simulink model "Control_Logic_b_chk2"  (R2019b)
settings: Solver=VariableStepAuto  StartTime=Start_time  StopTime=Stop_time  RelTol=1e-3
values from neighbouring files (symbols this model uses):
  Aset_N1 = 2    [Parameter_control.m]
  Aset_N10 = -10    [Parameter_control.m]
  Aset_N11 = 10    [Parameter_control.m]
  Aset_N12 = 20    [Parameter_control.m]
  Aset_N2 = 30    [Parameter_control.m]
  Aset_N3 = 3    [Parameter_control.m]
  Aset_N4 = 5    [Parameter_control.m]
  Aset_N5 = 1    [Parameter_control.m]
  Aset_N6 = 0    [Parameter_control.m]
  Aset_N7 = 0.01    [Parameter_control.m]
  Aset_N8 = 2    [Parameter_control.m]
  Aset_N9 = 0.1    [Parameter_control.m]
  Dset_N1 = 1    [Parameter_control.m]
  Dset_N2 = 1    [Parameter_control.m]
  Sample_time = 0.1    [main.m]    (also in test_tool_initialize.m)
undefined symbols (not defined in the file or in its folder): DiscIntNeverNeededParam
(part 2 of 3)

== system Control_Logic_b_chk2/OSHOTC5 ==
  In1 : Inport
  In2 : Inport  Port=2
  In3 : Inport  Port=3
  Data Type Conversion : DataTypeConversion  OutDataTypeStr=boolean
  MATLAB Function : MATLAB Function  TreatAsAtomicUnit=on  SystemSampleTime=Sample_time
  Memory : Memory  InheritSampleTime=on
  Memory1 : Memory  InheritSampleTime=on  LinearizeAsDelay=on
  Mux : Mux  Inputs=2
  Out1 : Outport  VectorParamsAs1DForOutWhenUnconnected=off
  wires:
  Memory/1 -> Mux/2
  MATLAB Function/1(y) -> Out1/1, Memory1/1
  In2/1 -> MATLAB Function/3(set)
  Mux/1 -> MATLAB Function/4(timc)
  In1/1 -> MATLAB Function/1(u)
  Memory1/1 -> Data Type Conversion/1
  Data Type Conversion/1 -> MATLAB Function/2(yold)
  MATLAB Function/2(w) -> Memory/1
  In3/1 -> Mux/1

== system Control_Logic_b_chk2/OSHOTC6 ==
  In1 : Inport
  In2 : Inport  Port=2
  In3 : Inport  Port=3
  Data Type Conversion : DataTypeConversion  OutDataTypeStr=boolean
  MATLAB Function : MATLAB Function  TreatAsAtomicUnit=on  SystemSampleTime=Sample_time
  Memory : Memory  InheritSampleTime=on
  Memory1 : Memory  InheritSampleTime=on  LinearizeAsDelay=on
  Mux : Mux  Inputs=2
  Out1 : Outport  VectorParamsAs1DForOutWhenUnconnected=off
  wires:
  Memory/1 -> Mux/2
  MATLAB Function/1(y) -> Out1/1, Memory1/1
  In2/1 -> MATLAB Function/3(set)
  Mux/1 -> MATLAB Function/4(timc)
  In1/1 -> MATLAB Function/1(u)
  Memory1/1 -> Data Type Conversion/1
  Data Type Conversion/1 -> MATLAB Function/2(yold)
  MATLAB Function/2(w) -> Memory/1
  In3/1 -> Mux/1

== system Control_Logic_b_chk2/OSHOTC7 ==
  In1 : Inport
  In2 : Inport  Port=2
  In3 : Inport  Port=3
  Data Type Conversion : DataTypeConversion  OutDataTypeStr=boolean
  MATLAB Function : MATLAB Function  TreatAsAtomicUnit=on  SystemSampleTime=Sample_time
  Memory : Memory  InheritSampleTime=on
  Memory1 : Memory  InheritSampleTime=on  LinearizeAsDelay=on
  Mux : Mux  Inputs=2
  Out1 : Outport  VectorParamsAs1DForOutWhenUnconnected=off
  wires:
  Memory/1 -> Mux/2
  MATLAB Function/1(y) -> Out1/1, Memory1/1
  In2/1 -> MATLAB Function/3(set)
  Mux/1 -> MATLAB Function/4(timc)
  In1/1 -> MATLAB Function/1(u)
  Memory1/1 -> Data Type Conversion/1
  Data Type Conversion/1 -> MATLAB Function/2(yold)
  MATLAB Function/2(w) -> Memory/1
  In3/1 -> Mux/1

== system Control_Logic_b_chk2/OSHOTC8 ==
  In1 : Inport
  In2 : Inport  Port=2
  In3 : Inport  Port=3
  Data Type Conversion : DataTypeConversion  OutDataTypeStr=boolean
  MATLAB Function : MATLAB Function  TreatAsAtomicUnit=on  SystemSampleTime=Sample_time
  Memory : Memory  InheritSampleTime=on
  Memory1 : Memory  InheritSampleTime=on  LinearizeAsDelay=on
  Mux : Mux  Inputs=2
  Out1 : Outport  VectorParamsAs1DForOutWhenUnconnected=off
  wires:
  Memory/1 -> Mux/2
  MATLAB Function/1(y) -> Out1/1, Memory1/1
  In2/1 -> MATLAB Function/3(set)
  Mux/1 -> MATLAB Function/4(timc)
  In1/1 -> MATLAB Function/1(u)
  Memory1/1 -> Data Type Conversion/1
  Data Type Conversion/1 -> MATLAB Function/2(yold)
  MATLAB Function/2(w) -> Memory/1
  In3/1 -> Mux/1

== system Control_Logic_b_chk2/OSHOTC9 ==
  In1 : Inport
  In2 : Inport  Port=2
  In3 : Inport  Port=3
  Data Type Conversion : DataTypeConversion  OutDataTypeStr=boolean
  MATLAB Function : MATLAB Function  TreatAsAtomicUnit=on  SystemSampleTime=Sample_time
  Memory : Memory  InheritSampleTime=on
  Memory1 : Memory  InheritSampleTime=on  LinearizeAsDelay=on
  Mux : Mux  Inputs=2
  Out1 : Outport  VectorParamsAs1DForOutWhenUnconnected=off
  wires:
  Memory/1 -> Mux/2
  MATLAB Function/1(y) -> Out1/1, Memory1/1
  In2/1 -> MATLAB Function/3(set)
  Mux/1 -> MATLAB Function/4(timc)
  In1/1 -> MATLAB Function/1(u)
  Memory1/1 -> Data Type Conversion/1
  Data Type Conversion/1 -> MATLAB Function/2(yold)
  MATLAB Function/2(w) -> Memory/1
  In3/1 -> Mux/1

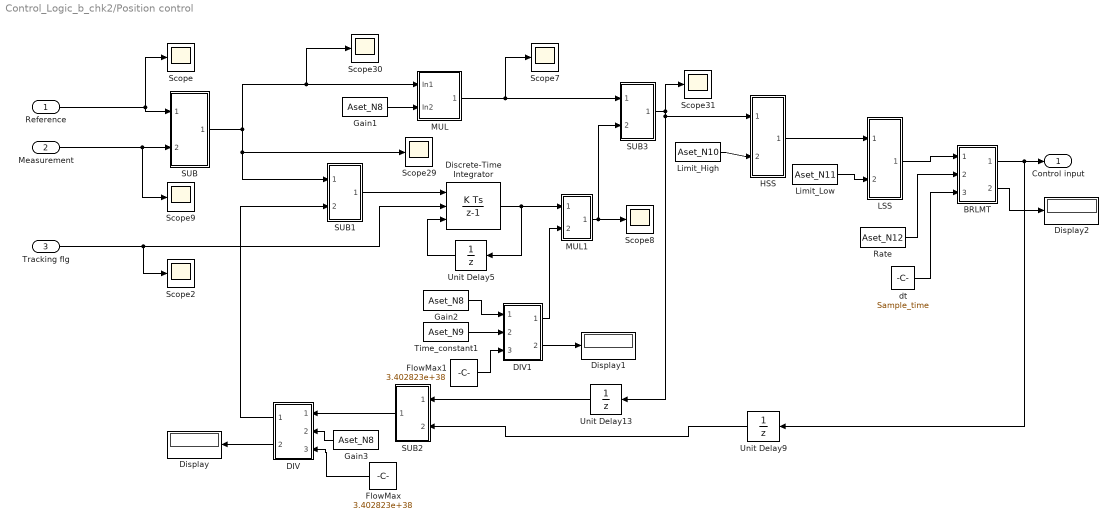
== system Control_Logic_b_chk2/Position control ==
  Reference : Inport
  Measurement : Inport  Port=2
  Tracking flg : Inport  Port=3
  BRLMT : Subsystem
  DIV : Subsystem
  DIV1 : Subsystem
  Discrete-Time Integrator : DiscreteIntegrator  ExternalReset=level  InitialConditionSource=external  SampleTime=Sample_time  ICPrevOutput=DiscIntNeverNeededParam  ICPrevScaledInput=DiscIntNeverNeededParam
  Display : Display
  Display1 : Display
  Display2 : Display
  FlowMax : Constant  Value=3.402823e+38  OutDataTypeStr=double  SampleTime=Sample_time
  FlowMax1 : Constant  Value=3.402823e+38  OutDataTypeStr=double  SampleTime=Sample_time
  Gain1 : Constant  Value=Aset_N8  OutDataTypeStr=double  SampleTime=Sample_time
  Gain2 : Constant  Value=Aset_N8  OutDataTypeStr=double  SampleTime=Sample_time
  Gain3 : Constant  Value=Aset_N8  OutDataTypeStr=double  SampleTime=Sample_time
  HSS : Subsystem
  LSS : Subsystem
  Limit_High : Constant  Value=Aset_N10  OutDataTypeStr=double  SampleTime=Sample_time
  Limit_Low : Constant  Value=Aset_N11  OutDataTypeStr=double  SampleTime=Sample_time
  MUL : Subsystem
  MUL1 : Subsystem
  Rate : Constant  Value=Aset_N12  OutDataTypeStr=double  SampleTime=Sample_time
  SUB : Subsystem
  SUB1 : Subsystem
  SUB2 : Subsystem
  SUB3 : Subsystem
  Scope{,2,7..9,29..31} (8 alike) : Scope
  Time_constant1 : Constant  Value=Aset_N9  OutDataTypeStr=double  SampleTime=Sample_time
  Unit Delay13 : UnitDelay  SampleTime=Sample_time  HasFrameUpgradeWarning=on
  Unit Delay5 : UnitDelay  SampleTime=Sample_time  HasFrameUpgradeWarning=on
  Unit Delay9 : UnitDelay  SampleTime=Sample_time  HasFrameUpgradeWarning=on
  dt : Constant  Value=Sample_time  OutDataTypeStr=double  SampleTime=Sample_time
  Control input : Outport  VectorParamsAs1DForOutWhenUnconnected=off
  wires:
  SUB3/1(Out1) -> Unit Delay13/1, HSS/1(In1), Scope31/1
  Measurement/1 -> Scope9/1, SUB/2(In2)
  SUB/1(Out1) -> Scope30/1, MUL/1(In1), SUB1/1(In1), Scope29/1
  DIV1/1(Out1) -> MUL1/2(In2)
  Unit Delay13/1 -> SUB2/1(In1)
  MUL/1(Out1) -> SUB3/1(In1), Scope7/1
  SUB2/1(Out1) -> DIV/1(In1)
  SUB1/1(Out1) -> Discrete-Time Integrator/1
  Gain1/1 -> MUL/2(In2)
  LSS/1(Out1) -> BRLMT/1(In1)
  Reference/1 -> SUB/1(In1), Scope/1
  Gain3/1 -> DIV/2(In2)
  Limit_Low/1 -> LSS/2(In2)
  Unit Delay5/1 -> Discrete-Time Integrator/3
  Tracking flg/1 -> Scope2/1, Discrete-Time Integrator/2
  Discrete-Time Integrator/1 -> MUL1/1(In1), Unit Delay5/1
  Limit_High/1 -> HSS/2(In2)
  MUL1/1(Out1) -> SUB3/2(In2), Scope8/1
  BRLMT/1(Out1) -> Control input/1, Unit Delay9/1
  Time_constant1/1 -> DIV1/2(In2)
  Gain2/1 -> DIV1/1(In1)
  HSS/1(Out1) -> LSS/1(In1)
  DIV/1(Out1) -> SUB1/2(In2)
  Unit Delay9/1 -> SUB2/2(In2)
  FlowMax/1 -> DIV/3(In3)
  DIV/2(Out2) -> Display/1
  FlowMax1/1 -> DIV1/3(In3)
  DIV1/2(Out2) -> Display1/1
  dt/1 -> BRLMT/3(In3)
  Rate/1 -> BRLMT/2(In2)
  BRLMT/2(Out2) -> Display2/1

== system Control_Logic_b_chk2/SUB ==
  In1 : Inport
  In2 : Inport  Port=2
  MATLAB Function : MATLAB Function  TreatAsAtomicUnit=on  SystemSampleTime=Sample_time
  Mux : Mux  Inputs=2
  Out1 : Outport  VectorParamsAs1DForOutWhenUnconnected=off
  wires:
  In2/1 -> Mux/2
  MATLAB Function/1(y) -> Out1/1
  Mux/1 -> MATLAB Function/1(u)
  In1/1 -> Mux/1

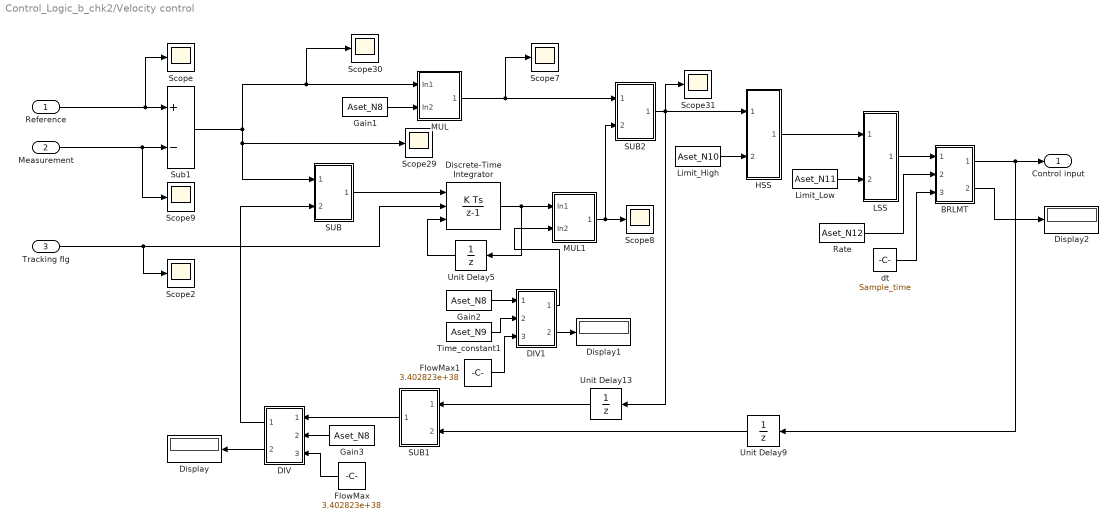
== system Control_Logic_b_chk2/Velocity control ==
  Reference : Inport
  Measurement : Inport  Port=2
  Tracking flg : Inport  Port=3
  BRLMT : Subsystem
  DIV : Subsystem
  DIV1 : Subsystem
  Discrete-Time Integrator : DiscreteIntegrator  ExternalReset=level  InitialConditionSource=external  SampleTime=Sample_time  ICPrevOutput=DiscIntNeverNeededParam  ICPrevScaledInput=DiscIntNeverNeededParam
  Display : Display
  Display1 : Display
  Display2 : Display
  FlowMax : Constant  Value=3.402823e+38  OutDataTypeStr=double  SampleTime=Sample_time
  FlowMax1 : Constant  Value=3.402823e+38  OutDataTypeStr=double  SampleTime=Sample_time
  Gain1 : Constant  Value=Aset_N8  OutDataTypeStr=double  SampleTime=Sample_time
  Gain2 : Constant  Value=Aset_N8  OutDataTypeStr=double  SampleTime=Sample_time
  Gain3 : Constant  Value=Aset_N8  OutDataTypeStr=double  SampleTime=Sample_time
  HSS : Subsystem
  LSS : Subsystem
  Limit_High : Constant  Value=Aset_N10  OutDataTypeStr=double  SampleTime=Sample_time
  Limit_Low : Constant  Value=Aset_N11  OutDataTypeStr=double  SampleTime=Sample_time
  MUL : Subsystem
  MUL1 : Subsystem
  Rate : Constant  Value=Aset_N12  OutDataTypeStr=double  SampleTime=Sample_time
  SUB : Subsystem
  SUB1 : Subsystem
  SUB2 : Subsystem
  Scope{,2,7..9,29..31} (8 alike) : Scope
  Sub1 : Sum  Inputs=+-  OutDataTypeStr=double
  Time_constant1 : Constant  Value=Aset_N9  OutDataTypeStr=double  SampleTime=Sample_time
  Unit Delay13 : UnitDelay  SampleTime=Sample_time  HasFrameUpgradeWarning=on
  Unit Delay5 : UnitDelay  SampleTime=Sample_time  HasFrameUpgradeWarning=on
  Unit Delay9 : UnitDelay  SampleTime=Sample_time  HasFrameUpgradeWarning=on
  dt : Constant  Value=Sample_time  OutDataTypeStr=double  SampleTime=Sample_time
  Control input : Outport  VectorParamsAs1DForOutWhenUnconnected=off
  wires:
  Unit Delay9/1 -> SUB1/2(In2)
  DIV/1(Out1) -> SUB/2(In2)
  HSS/1(Out1) -> LSS/1(In1)
  Gain2/1 -> DIV1/1(In1)
  Time_constant1/1 -> DIV1/2(In2)
  BRLMT/1(Out1) -> Control input/1, Unit Delay9/1
  MUL1/1(Out1) -> Scope8/1, SUB2/2(In2)
  Limit_High/1 -> HSS/2(In2)
  Discrete-Time Integrator/1 -> MUL1/1(In1), Unit Delay5/1
  Tracking flg/1 -> Discrete-Time Integrator/2, Scope2/1
  Unit Delay5/1 -> Discrete-Time Integrator/3
  Limit_Low/1 -> LSS/2(In2)
  Gain3/1 -> DIV/2(In2)
  Reference/1 -> Sub1/1, Scope/1
  LSS/1(Out1) -> BRLMT/1(In1)
  Gain1/1 -> MUL/2(In2)
  SUB/1(Out1) -> Discrete-Time Integrator/1
  SUB1/1(Out1) -> DIV/1(In1)
  MUL/1(Out1) -> SUB2/1(In1), Scope7/1
  Unit Delay13/1 -> SUB1/1(In1)
  DIV1/1(Out1) -> MUL1/2(In2)
  Sub1/1 -> SUB/1(In1), Scope29/1, MUL/1(In1), Scope30/1
  Measurement/1 -> Sub1/2, Scope9/1
  SUB2/1(Out1) -> HSS/1(In1), Scope31/1, Unit Delay13/1
  FlowMax/1 -> DIV/3(In3)
  DIV/2(Out2) -> Display/1
  DIV1/2(Out2) -> Display1/1
  FlowMax1/1 -> DIV1/3(In3)
  dt/1 -> BRLMT/3(In3)
  BRLMT/2(Out2) -> Display2/1
  Rate/1 -> BRLMT/2(In2)

== system Control_Logic_b_chk2/Position control/BRLMT ==
  In1 : Inport
  In2 : Inport  Port=2
  In3 : Inport  Port=3
  MATLAB Function : MATLAB Function  TreatAsAtomicUnit=on  SystemSampleTime=Sample_time
  Memory : Memory  InheritSampleTime=on
  Mux : Mux  Inputs=2
  Out1 : Outport  VectorParamsAs1DForOutWhenUnconnected=off
  Out2 : Outport  Port=2  VectorParamsAs1DForOutWhenUnconnected=off
  wires:
  In3/1 -> Mux/2
  In2/1 -> Mux/1
  Mux/1 -> MATLAB Function/3(set)
  MATLAB Function/2(delta) -> Out2/1
  Memory/1 -> MATLAB Function/2(yold)
  MATLAB Function/1(y) -> Out1/1, Memory/1
  In1/1 -> MATLAB Function/1(u)

== system Control_Logic_b_chk2/Position control/DIV ==
  In1 : Inport
  In2 : Inport  Port=2
  In3 : Inport  Port=3
  MATLAB Function : MATLAB Function  TreatAsAtomicUnit=on  SystemSampleTime=Sample_time
  Mux : Mux  Inputs=2
  Out1 : Outport  VectorParamsAs1DForOutWhenUnconnected=off
  Out2 : Outport  Port=2  VectorParamsAs1DForOutWhenUnconnected=off
  wires:
  In2/1 -> Mux/2
  In3/1 -> MATLAB Function/2(set)
  Mux/1 -> MATLAB Function/1(u)
  MATLAB Function/1(y) -> Out1/1
  MATLAB Function/2(err) -> Out2/1
  In1/1 -> Mux/1

== system Control_Logic_b_chk2/Position control/DIV1 ==
  In1 : Inport
  In2 : Inport  Port=2
  In3 : Inport  Port=3
  MATLAB Function : MATLAB Function  TreatAsAtomicUnit=on  SystemSampleTime=Sample_time
  Mux : Mux  Inputs=2
  Out1 : Outport  VectorParamsAs1DForOutWhenUnconnected=off
  Out2 : Outport  Port=2  VectorParamsAs1DForOutWhenUnconnected=off
  wires:
  In2/1 -> Mux/2
  In3/1 -> MATLAB Function/2(set)
  Mux/1 -> MATLAB Function/1(u)
  MATLAB Function/1(y) -> Out1/1
  MATLAB Function/2(err) -> Out2/1
  In1/1 -> Mux/1

== system Control_Logic_b_chk2/Position control/HSS ==
  In1 : Inport
  In2 : Inport  Port=2
  MATLAB Function : MATLAB Function  TreatAsAtomicUnit=on
  Mux : Mux  Inputs=2
  Out1 : Outport  VectorParamsAs1DForOutWhenUnconnected=off
  wires:
  Mux/1 -> MATLAB Function/1(u)
  In1/1 -> Mux/1
  MATLAB Function/1(y) -> Out1/1
  In2/1 -> Mux/2

== system Control_Logic_b_chk2/Position control/LSS ==
  In1 : Inport
  In2 : Inport  Port=2
  MATLAB Function : MATLAB Function  TreatAsAtomicUnit=on  SystemSampleTime=Sample_time
  Mux : Mux  Inputs=2
  Out1 : Outport  VectorParamsAs1DForOutWhenUnconnected=off
  wires:
  MATLAB Function/1(y) -> Out1/1
  Mux/1 -> MATLAB Function/1(u)
  In1/1 -> Mux/1
  In2/1 -> Mux/2

== system Control_Logic_b_chk2/Position control/MUL ==
  In1 : Inport
  In2 : Inport  Port=2
  MATLAB Function : MATLAB Function  TreatAsAtomicUnit=on  SystemSampleTime=Sample_time
  Mux : Mux  Inputs=2
  Out1 : Outport  VectorParamsAs1DForOutWhenUnconnected=off
  wires:
  Mux/1 -> MATLAB Function/1(u)
  In1/1 -> Mux/1
  In2/1 -> Mux/2
  MATLAB Function/1(y) -> Out1/1

== system Control_Logic_b_chk2/Position control/MUL1 ==
  In1 : Inport
  In2 : Inport  Port=2
  MATLAB Function : MATLAB Function  TreatAsAtomicUnit=on  SystemSampleTime=Sample_time
  Mux : Mux  Inputs=2
  Out1 : Outport  VectorParamsAs1DForOutWhenUnconnected=off
  wires:
  Mux/1 -> MATLAB Function/1(u)
  In1/1 -> Mux/1
  In2/1 -> Mux/2
  MATLAB Function/1(y) -> Out1/1

== system Control_Logic_b_chk2/Position control/SUB ==
  In1 : Inport
  In2 : Inport  Port=2
  MATLAB Function : MATLAB Function  TreatAsAtomicUnit=on  SystemSampleTime=Sample_time
  Mux : Mux  Inputs=2
  Out1 : Outport  VectorParamsAs1DForOutWhenUnconnected=off
  wires:
  In2/1 -> Mux/2
  MATLAB Function/1(y) -> Out1/1
  Mux/1 -> MATLAB Function/1(u)
  In1/1 -> Mux/1

== system Control_Logic_b_chk2/Position control/SUB1 ==
  In1 : Inport
  In2 : Inport  Port=2
  MATLAB Function : MATLAB Function  TreatAsAtomicUnit=on  SystemSampleTime=Sample_time
  Mux : Mux  Inputs=2
  Out1 : Outport  VectorParamsAs1DForOutWhenUnconnected=off
  wires:
  In2/1 -> Mux/2
  MATLAB Function/1(y) -> Out1/1
  Mux/1 -> MATLAB Function/1(u)
  In1/1 -> Mux/1

== system Control_Logic_b_chk2/Position control/SUB2 ==
  In1 : Inport
  In2 : Inport  Port=2
  MATLAB Function : MATLAB Function  TreatAsAtomicUnit=on  SystemSampleTime=Sample_time
  Mux : Mux  Inputs=2
  Out1 : Outport  VectorParamsAs1DForOutWhenUnconnected=off
  wires:
  In2/1 -> Mux/2
  MATLAB Function/1(y) -> Out1/1
  Mux/1 -> MATLAB Function/1(u)
  In1/1 -> Mux/1

== system Control_Logic_b_chk2/Position control/SUB3 ==
  In1 : Inport
  In2 : Inport  Port=2
  MATLAB Function : MATLAB Function  TreatAsAtomicUnit=on  SystemSampleTime=Sample_time
  Mux : Mux  Inputs=2
  Out1 : Outport  VectorParamsAs1DForOutWhenUnconnected=off
  wires:
  In2/1 -> Mux/2
  MATLAB Function/1(y) -> Out1/1
  Mux/1 -> MATLAB Function/1(u)
  In1/1 -> Mux/1

== system Control_Logic_b_chk2/Velocity control/BRLMT ==
  In1 : Inport
  In2 : Inport  Port=2
  In3 : Inport  Port=3
  MATLAB Function : MATLAB Function  TreatAsAtomicUnit=on  SystemSampleTime=Sample_time
  Memory : Memory  InheritSampleTime=on
  Mux : Mux  Inputs=2
  Out1 : Outport  VectorParamsAs1DForOutWhenUnconnected=off
  Out2 : Outport  Port=2  VectorParamsAs1DForOutWhenUnconnected=off
  wires:
  In3/1 -> Mux/2
  In2/1 -> Mux/1
  Mux/1 -> MATLAB Function/3(set)
  MATLAB Function/2(delta) -> Out2/1
  Memory/1 -> MATLAB Function/2(yold)
  MATLAB Function/1(y) -> Out1/1, Memory/1
  In1/1 -> MATLAB Function/1(u)

== system Control_Logic_b_chk2/Velocity control/DIV ==
  In1 : Inport
  In2 : Inport  Port=2
  In3 : Inport  Port=3
  MATLAB Function : MATLAB Function  TreatAsAtomicUnit=on  SystemSampleTime=Sample_time
  Mux : Mux  Inputs=2
  Out1 : Outport  VectorParamsAs1DForOutWhenUnconnected=off
  Out2 : Outport  Port=2  VectorParamsAs1DForOutWhenUnconnected=off
  wires:
  In2/1 -> Mux/2
  In3/1 -> MATLAB Function/2(set)
  Mux/1 -> MATLAB Function/1(u)
  MATLAB Function/1(y) -> Out1/1
  MATLAB Function/2(err) -> Out2/1
  In1/1 -> Mux/1

== system Control_Logic_b_chk2/Velocity control/DIV1 ==
  In1 : Inport
  In2 : Inport  Port=2
  In3 : Inport  Port=3
  MATLAB Function : MATLAB Function  TreatAsAtomicUnit=on  SystemSampleTime=Sample_time
  Mux : Mux  Inputs=2
  Out1 : Outport  VectorParamsAs1DForOutWhenUnconnected=off
  Out2 : Outport  Port=2  VectorParamsAs1DForOutWhenUnconnected=off
  wires:
  In2/1 -> Mux/2
  In3/1 -> MATLAB Function/2(set)
  Mux/1 -> MATLAB Function/1(u)
  MATLAB Function/1(y) -> Out1/1
  MATLAB Function/2(err) -> Out2/1
  In1/1 -> Mux/1

== system Control_Logic_b_chk2/Velocity control/HSS ==
  In1 : Inport
  In2 : Inport  Port=2
  MATLAB Function : MATLAB Function  TreatAsAtomicUnit=on
  Mux : Mux  Inputs=2
  Out1 : Outport  VectorParamsAs1DForOutWhenUnconnected=off
  wires:
  Mux/1 -> MATLAB Function/1(u)
  In1/1 -> Mux/1
  MATLAB Function/1(y) -> Out1/1
  In2/1 -> Mux/2

== system Control_Logic_b_chk2/Velocity control/LSS ==
  In1 : Inport
  In2 : Inport  Port=2
  MATLAB Function : MATLAB Function  TreatAsAtomicUnit=on  SystemSampleTime=Sample_time
  Mux : Mux  Inputs=2
  Out1 : Outport  VectorParamsAs1DForOutWhenUnconnected=off
  wires:
  MATLAB Function/1(y) -> Out1/1
  Mux/1 -> MATLAB Function/1(u)
  In1/1 -> Mux/1
  In2/1 -> Mux/2

== system Control_Logic_b_chk2/Velocity control/MUL ==
  In1 : Inport
  In2 : Inport  Port=2
  MATLAB Function : MATLAB Function  TreatAsAtomicUnit=on  SystemSampleTime=Sample_time
  Mux : Mux  Inputs=2
  Out1 : Outport  VectorParamsAs1DForOutWhenUnconnected=off
  wires:
  Mux/1 -> MATLAB Function/1(u)
  In1/1 -> Mux/1
  In2/1 -> Mux/2
  MATLAB Function/1(y) -> Out1/1

== system Control_Logic_b_chk2/Velocity control/MUL1 ==
  In1 : Inport
  In2 : Inport  Port=2
  MATLAB Function : MATLAB Function  TreatAsAtomicUnit=on  SystemSampleTime=Sample_time
  Mux : Mux  Inputs=2
  Out1 : Outport  VectorParamsAs1DForOutWhenUnconnected=off
  wires:
  Mux/1 -> MATLAB Function/1(u)
  In1/1 -> Mux/1
  In2/1 -> Mux/2
  MATLAB Function/1(y) -> Out1/1

== system Control_Logic_b_chk2/Velocity control/SUB ==
  In1 : Inport
  In2 : Inport  Port=2
  MATLAB Function : MATLAB Function  TreatAsAtomicUnit=on  SystemSampleTime=Sample_time
  Mux : Mux  Inputs=2
  Out1 : Outport  VectorParamsAs1DForOutWhenUnconnected=off
  wires:
  In2/1 -> Mux/2
  MATLAB Function/1(y) -> Out1/1
  Mux/1 -> MATLAB Function/1(u)
  In1/1 -> Mux/1

== system Control_Logic_b_chk2/Velocity control/SUB1 ==
  In1 : Inport
  In2 : Inport  Port=2
  MATLAB Function : MATLAB Function  TreatAsAtomicUnit=on  SystemSampleTime=Sample_time
  Mux : Mux  Inputs=2
  Out1 : Outport  VectorParamsAs1DForOutWhenUnconnected=off
  wires:
  In2/1 -> Mux/2
  MATLAB Function/1(y) -> Out1/1
  Mux/1 -> MATLAB Function/1(u)
  In1/1 -> Mux/1

== system Control_Logic_b_chk2/Velocity control/SUB2 ==
  In1 : Inport
  In2 : Inport  Port=2
  MATLAB Function : MATLAB Function  TreatAsAtomicUnit=on  SystemSampleTime=Sample_time
  Mux : Mux  Inputs=2
  Out1 : Outport  VectorParamsAs1DForOutWhenUnconnected=off
  wires:
  In2/1 -> Mux/2
  MATLAB Function/1(y) -> Out1/1
  Mux/1 -> MATLAB Function/1(u)
  In1/1 -> Mux/1

== matlab function Control_Logic_b_chk2/HLM/MATLAB Function ==
  data: u input; y output; set input
% 高低モニタ
%   x＞高側設定値ならば、 yをON
%   x＜低側設定値ならば、 yをON
%   上記以外ならばyをOFF
%       u :入力変数
%       set(1)：低側設定値
%       set(2)：高側設定値
%       y : 出力変数
function y = HLM(u, set)
    if (u > set(1)) || (u < set(2))
        y= true;
    else
        y = false; 
    end

== matlab function Control_Logic_b_chk2/ABS/MATLAB Function ==
  data: u input; y output
% 絶対値
function y = ABS(u)
    if u > 0
        y = u;
    else
        y = -u;
    end

== matlab function Control_Logic_b_chk2/NOT/MATLAB Function ==
  data: u input; y output
%反転
function y = NOT(u)
    if u == false        
        y = true;
    else
        y = false;
    end

== matlab function Control_Logic_b_chk2/NOT1/MATLAB Function ==
  data: u input; y output
%反転
function y = NOT(u)
    if u == false        
        y = true;
    else
        y = false;
    end

== matlab function Control_Logic_b_chk2/OFDLC/MATLAB Function ==
  data: ud input; set input; y output; w output; timc input
% オフディレイ タイマ
%  xがOFFとなってからパラメータで設定した[sec]後にyがOFFとなる。
%  なお、xのOFF状態がパラメータで設定した[sec]続かずにON状態
%  へ戻った場合はyはON状態を継続する。
%       ud:入力信号
%       set：時定数
%       timc(1)：計算刻み
%       timc(2)：経過時間(前回値)
%       y : 出力信号
function[y, w] = OFDLC(ud, set, timc)
    if ud == true
        y = true; 
        w = set;
    else
        if timc(2) > 0 
            y = true;
            w = timc(2) - timc(1);
        else
            y = false;
            w = timc(2);
        end
    end

== matlab function Control_Logic_b_chk2/OFDLC1/MATLAB Function ==
  data: ud input; set input; y output; w output; timc input
% オフディレイ タイマ
%  xがOFFとなってからパラメータで設定した[sec]後にyがOFFとなる。
%  なお、xのOFF状態がパラメータで設定した[sec]続かずにON状態
%  へ戻った場合はyはON状態を継続する。
%       ud:入力信号
%       set：時定数
%       timc(1)：計算刻み
%       timc(2)：経過時間(前回値)
%       y : 出力信号
function[y, w] = OFDLC(ud, set, timc)
    if ud == true
        y = true; 
        w = set;
    else
        if timc(2) > 0 
            y = true;
            w = timc(2) - timc(1);
        else
            y = false;
            w = timc(2);
        end
    end

== matlab function Control_Logic_b_chk2/AND3L/MATLAB Function ==
  data: u input; y output
% 論理積
function y = AND3(u)
    y = u(1) & u(2) & u(3);

== matlab function Control_Logic_b_chk2/AND3L1/MATLAB Function ==
  data: u input; y output
% 論理積
function y = AND3(u)
    y = u(1) & u(2) & u(3);

== matlab function Control_Logic_b_chk2/AND/MATLAB Function ==
  data: u input; y output
% 論理積
function y = AND(u)
    y = u(1) & u(2);

== matlab function Control_Logic_b_chk2/AND1/MATLAB Function ==
  data: u input; y output
% 論理積
function y = AND(u)
    y = u(1) & u(2);

== matlab function Control_Logic_b_chk2/ONDLC/MATLAB Function ==
  data: ud input; set input; y output; w output; timc input
% オンディレイ タイマ
%  xがONとなってからパラメータで設定した[sec]後にyがONとなる。
%  なお、xのON状態がパラメータで設定した[sec]続かずにOFF状態
%  へ戻った場合はyはOFF状態を継続する。
%       ud :入力信号
%       set：時定数
%       timc(1)：計算刻み
%       timc(2)：経過時間(前回値)
%       y : 出力信号
function [y, w] = ONDLC(ud, set, timc)
    if ud == false
        y = false;
        w = 0;
    else
        if timc(2) < set 
            y = false;
            w = timc(2) + timc(1);
        else
            y = true;
            w = timc(2);
        end
    end

== matlab function Control_Logic_b_chk2/FF/MATLAB Function ==
  data: yold input; y output; set input
% フリップフロップ
%  セット入力がONのとき、yはON
%  リセット入力がONのとき、yはOFF
%  セット入力、リセット入力共にONまたはOFFのときは前回値を保持
%       yold:前回値
%       set(1):セット信号
%       set(2)：リセット信号
%       y : 出力信号
function y = FF(yold, set)
    y = yold;
    if (set(1) == false) && (set(2) == true)
        y = false;
    else
        if (set(1) == true) && (set(2) == false)
            y = true;
        end
    end

== matlab function Control_Logic_b_chk2/OFDLC2/MATLAB Function ==
  data: ud input; set input; y output; w output; timc input
% オフディレイ タイマ
%  xがOFFとなってからパラメータで設定した[sec]後にyがOFFとなる。
%  なお、xのOFF状態がパラメータで設定した[sec]続かずにON状態
%  へ戻った場合はyはON状態を継続する。
%       ud:入力信号
%       set：時定数
%       timc(1)：計算刻み
%       timc(2)：経過時間(前回値)
%       y : 出力信号
function[y, w] = OFDLC(ud, set, timc)
    if ud == true
        y = true; 
        w = set;
    else
        if timc(2) > 0 
            y = true;
            w = timc(2) - timc(1);
        else
            y = false;
            w = timc(2);
        end
    end

== matlab function Control_Logic_b_chk2/OFDLC3/MATLAB Function ==
  data: ud input; set input; y output; w output; timc input
% オフディレイ タイマ
%  xがOFFとなってからパラメータで設定した[sec]後にyがOFFとなる。
%  なお、xのOFF状態がパラメータで設定した[sec]続かずにON状態
%  へ戻った場合はyはON状態を継続する。
%       ud:入力信号
%       set：時定数
%       timc(1)：計算刻み
%       timc(2)：経過時間(前回値)
%       y : 出力信号
function[y, w] = OFDLC(ud, set, timc)
    if ud == true
        y = true; 
        w = set;
    else
        if timc(2) > 0 
            y = true;
            w = timc(2) - timc(1);
        else
            y = false;
            w = timc(2);
        end
    end

== matlab function Control_Logic_b_chk2/OSHOTC/MATLAB Function ==
  data: u input; y output; w output; yold input; set input; timc input
% ワンショット タイマ
%  xがOFFからONに変化してからパラメータで設定した[sec]の間、yをONとする。
%  なお、xのON状態がパラメータで設定した[sec]以上継続した場合、あるいは設定以下
%  しか継続しない場合でも、yのON状態の期間はパラメータで設定した時間となる。
%       ud(1)：入力信号
%       yold：前回値
%       set：時定数
%       timc(1)：計算刻み
%       timc(2)：経過時間
%       y : 出力信号
function[y, w] = OSHOTC(u, yold, set, timc)
    if (u == false) && (yold == false)
        w = 0;
        y = false;
    else
        if set > timc(2)
            y = true;
            w = timc(2) + timc(1);
        else
            y = false;
            w = timc(2);
            if u == false
                w = 0;
            end
        end
    end

== matlab function Control_Logic_b_chk2/OSHOTC1/MATLAB Function ==
  data: u input; y output; w output; yold input; set input; timc input
% ワンショット タイマ
%  xがOFFからONに変化してからパラメータで設定した[sec]の間、yをONとする。
%  なお、xのON状態がパラメータで設定した[sec]以上継続した場合、あるいは設定以下
%  しか継続しない場合でも、yのON状態の期間はパラメータで設定した時間となる。
%       ud(1)：入力信号
%       yold：前回値
%       set：時定数
%       timc(1)：計算刻み
%       timc(2)：経過時間
%       y : 出力信号
function[y, w] = OSHOTC(u, yold, set, timc)
    if (u == false) && (yold == false)
        w = 0;
        y = false;
    else
        if set > timc(2)
            y = true;
            w = timc(2) + timc(1);
        else
            y = false;
            w = timc(2);
            if u == false
                w = 0;
            end
        end
    end

== matlab function Control_Logic_b_chk2/NOT2/MATLAB Function ==
  data: u input; y output
%反転
function y = NOT(u)
    if u == false        
        y = true;
    else
        y = false;
    end

== matlab function Control_Logic_b_chk2/NOT3/MATLAB Function ==
  data: u input; y output
%反転
function y = NOT(u)
    if u == false        
        y = true;
    else
        y = false;
    end

== matlab function Control_Logic_b_chk2/OR3L/MATLAB Function ==
  data: u input; y output
%論理和
function y = OR3(u)
    y = u(1) | u(2) | u(3);

== matlab function Control_Logic_b_chk2/ONDLC1/MATLAB Function ==
  data: ud input; set input; y output; w output; timc input
% オンディレイ タイマ
%  xがONとなってからパラメータで設定した[sec]後にyがONとなる。
%  なお、xのON状態がパラメータで設定した[sec]続かずにOFF状態
%  へ戻った場合はyはOFF状態を継続する。
%       ud :入力信号
%       set：時定数
%       timc(1)：計算刻み
%       timc(2)：経過時間(前回値)
%       y : 出力信号
function [y, w] = ONDLC(ud, set, timc)
    if ud == false
        y = false;
        w = 0;
    else
        if timc(2) < set 
            y = false;
            w = timc(2) + timc(1);
        else
            y = true;
            w = timc(2);
        end
    end

== matlab function Control_Logic_b_chk2/AND2/MATLAB Function ==
  data: u input; y output
% 論理積
function y = AND(u)
    y = u(1) & u(2);

== matlab function Control_Logic_b_chk2/FF1/MATLAB Function ==
  data: yold input; y output; set input
% フリップフロップ
%  セット入力がONのとき、yはON
%  リセット入力がONのとき、yはOFF
%  セット入力、リセット入力共にONまたはOFFのときは前回値を保持
%       yold:前回値
%       set(1):セット信号
%       set(2)：リセット信号
%       y : 出力信号
function y = FF(yold, set)
    y = yold;
    if (set(1) == false) && (set(2) == true)
        y = false;
    else
        if (set(1) == true) && (set(2) == false)
            y = true;
        end
    end

== matlab function Control_Logic_b_chk2/OR3L1/MATLAB Function ==
  data: u input; y output
%論理和
function y = OR3(u)
    y = u(1) | u(2) | u(3);

== matlab function Control_Logic_b_chk2/OR3L2/MATLAB Function ==
  data: u input; y output
%論理和
function y = OR3(u)
    y = u(1) | u(2) | u(3);

== matlab function Control_Logic_b_chk2/OSHOTC2/MATLAB Function ==
  data: u input; y output; w output; yold input; set input; timc input
% ワンショット タイマ
%  xがOFFからONに変化してからパラメータで設定した[sec]の間、yをONとする。
%  なお、xのON状態がパラメータで設定した[sec]以上継続した場合、あるいは設定以下
%  しか継続しない場合でも、yのON状態の期間はパラメータで設定した時間となる。
%       ud(1)：入力信号
%       yold：前回値
%       set：時定数
%       timc(1)：計算刻み
%       timc(2)：経過時間
%       y : 出力信号
function[y, w] = OSHOTC(u, yold, set, timc)
    if (u == false) && (yold == false)
        w = 0;
        y = false;
    else
        if set > timc(2)
            y = true;
            w = timc(2) + timc(1);
        else
            y = false;
            w = timc(2);
            if u == false
                w = 0;
            end
        end
    end

== matlab function Control_Logic_b_chk2/OSHOTC3/MATLAB Function ==
  data: u input; y output; w output; yold input; set input; timc input
% ワンショット タイマ
%  xがOFFからONに変化してからパラメータで設定した[sec]の間、yをONとする。
%  なお、xのON状態がパラメータで設定した[sec]以上継続した場合、あるいは設定以下
%  しか継続しない場合でも、yのON状態の期間はパラメータで設定した時間となる。
%       ud(1)：入力信号
%       yold：前回値
%       set：時定数
%       timc(1)：計算刻み
%       timc(2)：経過時間
%       y : 出力信号
function[y, w] = OSHOTC(u, yold, set, timc)
    if (u == false) && (yold == false)
        w = 0;
        y = false;
    else
        if set > timc(2)
            y = true;
            w = timc(2) + timc(1);
        else
            y = false;
            w = timc(2);
            if u == false
                w = 0;
            end
        end
    end

== matlab function Control_Logic_b_chk2/OSHOTC4/MATLAB Function ==
  data: u input; y output; w output; yold input; set input; timc input
% ワンショット タイマ
%  xがOFFからONに変化してからパラメータで設定した[sec]の間、yをONとする。
%  なお、xのON状態がパラメータで設定した[sec]以上継続した場合、あるいは設定以下
%  しか継続しない場合でも、yのON状態の期間はパラメータで設定した時間となる。
%       ud(1)：入力信号
%       yold：前回値
%       set：時定数
%       timc(1)：計算刻み
%       timc(2)：経過時間
%       y : 出力信号
function[y, w] = OSHOTC(u, yold, set, timc)
    if (u == false) && (yold == false)
        w = 0;
        y = false;
    else
        if set > timc(2)
            y = true;
            w = timc(2) + timc(1);
        else
            y = false;
            w = timc(2);
            if u == false
                w = 0;
            end
        end
    end

== matlab function Control_Logic_b_chk2/ONDLC2/MATLAB Function ==
  data: ud input; set input; y output; w output; timc input
% オンディレイ タイマ
%  xがONとなってからパラメータで設定した[sec]後にyがONとなる。
%  なお、xのON状態がパラメータで設定した[sec]続かずにOFF状態
%  へ戻った場合はyはOFF状態を継続する。
%       ud :入力信号
%       set：時定数
%       timc(1)：計算刻み
%       timc(2)：経過時間(前回値)
%       y : 出力信号
function [y, w] = ONDLC(ud, set, timc)
    if ud == false
        y = false;
        w = 0;
    else
        if timc(2) < set 
            y = false;
            w = timc(2) + timc(1);
        else
            y = true;
            w = timc(2);
        end
    end

== matlab function Control_Logic_b_chk2/AND3/MATLAB Function ==
  data: u input; y output
% 論理積
function y = AND(u)
    y = u(1) & u(2);

== matlab function Control_Logic_b_chk2/AND4/MATLAB Function ==
  data: u input; y output
% 論理積
function y = AND(u)
    y = u(1) & u(2);

== matlab function Control_Logic_b_chk2/OR3L3/MATLAB Function ==
  data: u input; y output
%論理和
function y = OR3(u)
    y = u(1) | u(2) | u(3);

== matlab function Control_Logic_b_chk2/AND5/MATLAB Function ==
  data: u input; y output
% 論理積
function y = AND(u)
    y = u(1) & u(2);

== matlab function Control_Logic_b_chk2/FF2/MATLAB Function ==
  data: yold input; y output; set input
% フリップフロップ
%  セット入力がONのとき、yはON
%  リセット入力がONのとき、yはOFF
%  セット入力、リセット入力共にONまたはOFFのときは前回値を保持
%       yold:前回値
%       set(1):セット信号
%       set(2)：リセット信号
%       y : 出力信号
function y = FF(yold, set)
    y = yold;
    if (set(1) == false) && (set(2) == true)
        y = false;
    else
        if (set(1) == true) && (set(2) == false)
            y = true;
        end
    end

== matlab function Control_Logic_b_chk2/OSHOTC5/MATLAB Function ==
  data: u input; y output; w output; yold input; set input; timc input
% ワンショット タイマ
%  xがOFFからONに変化してからパラメータで設定した[sec]の間、yをONとする。
%  なお、xのON状態がパラメータで設定した[sec]以上継続した場合、あるいは設定以下
%  しか継続しない場合でも、yのON状態の期間はパラメータで設定した時間となる。
%       ud(1)：入力信号
%       yold：前回値
%       set：時定数
%       timc(1)：計算刻み
%       timc(2)：経過時間
%       y : 出力信号
function[y, w] = OSHOTC(u, yold, set, timc)
    if (u == false) && (yold == false)
        w = 0;
        y = false;
    else
        if set > timc(2)
            y = true;
            w = timc(2) + timc(1);
        else
            y = false;
            w = timc(2);
            if u == false
                w = 0;
            end
        end
    end

== matlab function Control_Logic_b_chk2/OSHOTC6/MATLAB Function ==
  data: u input; y output; w output; yold input; set input; timc input
% ワンショット タイマ
%  xがOFFからONに変化してからパラメータで設定した[sec]の間、yをONとする。
%  なお、xのON状態がパラメータで設定した[sec]以上継続した場合、あるいは設定以下
%  しか継続しない場合でも、yのON状態の期間はパラメータで設定した時間となる。
%       ud(1)：入力信号
%       yold：前回値
%       set：時定数
%       timc(1)：計算刻み
%       timc(2)：経過時間
%       y : 出力信号
function[y, w] = OSHOTC(u, yold, set, timc)
    if (u == false) && (yold == false)
        w = 0;
        y = false;
    else
        if set > timc(2)
            y = true;
            w = timc(2) + timc(1);
        else
            y = false;
            w = timc(2);
            if u == false
                w = 0;
            end
        end
    end

== matlab function Control_Logic_b_chk2/OSHOTC7/MATLAB Function ==
  data: u input; y output; w output; yold input; set input; timc input
% ワンショット タイマ
%  xがOFFからONに変化してからパラメータで設定した[sec]の間、yをONとする。
%  なお、xのON状態がパラメータで設定した[sec]以上継続した場合、あるいは設定以下
%  しか継続しない場合でも、yのON状態の期間はパラメータで設定した時間となる。
%       ud(1)：入力信号
%       yold：前回値
%       set：時定数
%       timc(1)：計算刻み
%       timc(2)：経過時間
%       y : 出力信号
function[y, w] = OSHOTC(u, yold, set, timc)
    if (u == false) && (yold == false)
        w = 0;
        y = false;
    else
        if set > timc(2)
            y = true;
            w = timc(2) + timc(1);
        else
            y = false;
            w = timc(2);
            if u == false
                w = 0;
            end
        end
    end

== matlab function Control_Logic_b_chk2/OSHOTC8/MATLAB Function ==
  data: u input; y output; w output; yold input; set input; timc input
% ワンショット タイマ
%  xがOFFからONに変化してからパラメータで設定した[sec]の間、yをONとする。
%  なお、xのON状態がパラメータで設定した[sec]以上継続した場合、あるいは設定以下
%  しか継続しない場合でも、yのON状態の期間はパラメータで設定した時間となる。
%       ud(1)：入力信号
%       yold：前回値
%       set：時定数
%       timc(1)：計算刻み
%       timc(2)：経過時間
%       y : 出力信号
function[y, w] = OSHOTC(u, yold, set, timc)
    if (u == false) && (yold == false)
        w = 0;
        y = false;
    else
        if set > timc(2)
            y = true;
            w = timc(2) + timc(1);
        else
            y = false;
            w = timc(2);
            if u == false
                w = 0;
            end
        end
    end

== matlab function Control_Logic_b_chk2/OR3L4/MATLAB Function ==
  data: u input; y output
%論理和
function y = OR3(u)
    y = u(1) | u(2) | u(3);

== matlab function Control_Logic_b_chk2/OSHOTC9/MATLAB Function ==
  data: u input; y output; w output; yold input; set input; timc input
% ワンショット タイマ
%  xがOFFからONに変化してからパラメータで設定した[sec]の間、yをONとする。
%  なお、xのON状態がパラメータで設定した[sec]以上継続した場合、あるいは設定以下
%  しか継続しない場合でも、yのON状態の期間はパラメータで設定した時間となる。
%       ud(1)：入力信号
%       yold：前回値
%       set：時定数
%       timc(1)：計算刻み
%       timc(2)：経過時間
%       y : 出力信号
function[y, w] = OSHOTC(u, yold, set, timc)
    if (u == false) && (yold == false)
        w = 0;
        y = false;
    else
        if set > timc(2)
            y = true;
            w = timc(2) + timc(1);
        else
            y = false;
            w = timc(2);
            if u == false
                w = 0;
            end
        end
    end

== matlab function Control_Logic_b_chk2/OSHOTC10/MATLAB Function ==
  data: u input; y output; w output; yold input; set input; timc input
% ワンショット タイマ
%  xがOFFからONに変化してからパラメータで設定した[sec]の間、yをONとする。
%  なお、xのON状態がパラメータで設定した[sec]以上継続した場合、あるいは設定以下
%  しか継続しない場合でも、yのON状態の期間はパラメータで設定した時間となる。
%       ud(1)：入力信号
%       yold：前回値
%       set：時定数
%       timc(1)：計算刻み
%       timc(2)：経過時間
%       y : 出力信号
function[y, w] = OSHOTC(u, yold, set, timc)
    if (u == false) && (yold == false)
        w = 0;
        y = false;
    else
        if set > timc(2)
            y = true;
            w = timc(2) + timc(1);
        else
            y = false;
            w = timc(2);
            if u == false
                w = 0;
            end
        end
    end

== matlab function Control_Logic_b_chk2/OSHOTC11/MATLAB Function ==
  data: u input; y output; w output; yold input; set input; timc input
% ワンショット タイマ
%  xがOFFからONに変化してからパラメータで設定した[sec]の間、yをONとする。
%  なお、xのON状態がパラメータで設定した[sec]以上継続した場合、あるいは設定以下
%  しか継続しない場合でも、yのON状態の期間はパラメータで設定した時間となる。
%       ud(1)：入力信号
%       yold：前回値
%       set：時定数
%       timc(1)：計算刻み
%       timc(2)：経過時間
%       y : 出力信号
function[y, w] = OSHOTC(u, yold, set, timc)
    if (u == false) && (yold == false)
        w = 0;
        y = false;
    else
        if set > timc(2)
            y = true;
            w = timc(2) + timc(1);
        else
            y = false;
            w = timc(2);
            if u == false
                w = 0;
            end
        end
    end

== matlab function Control_Logic_b_chk2/NOT4/MATLAB Function ==
  data: u input; y output
%反転
function y = NOT(u)
    if u == false        
        y = true;
    else
        y = false;
    end

== matlab function Control_Logic_b_chk2/OR/MATLAB Function ==
  data: u input; y output
%論理和
function y = OR(u)
    y = u(1) | u(2);

== matlab function Control_Logic_b_chk2/AND6/MATLAB Function ==
  data: u input; y output
% 論理積
function y = AND(u)
    y = u(1) & u(2);

== matlab function Control_Logic_b_chk2/ONDLC3/MATLAB Function ==
  data: ud input; set input; y output; w output; timc input
% オンディレイ タイマ
%  xがONとなってからパラメータで設定した[sec]後にyがONとなる。
%  なお、xのON状態がパラメータで設定した[sec]続かずにOFF状態
%  へ戻った場合はyはOFF状態を継続する。
%       ud :入力信号
%       set：時定数
%       timc(1)：計算刻み
%       timc(2)：経過時間(前回値)
%       y : 出力信号
function [y, w] = ONDLC(ud, set, timc)
    if ud == false
        y = false;
        w = 0;
    else
        if timc(2) < set 
            y = false;
            w = timc(2) + timc(1);
        else
            y = true;
            w = timc(2);
        end
    end

== matlab function Control_Logic_b_chk2/OR1/MATLAB Function ==
  data: u input; y output
%論理和
function y = OR(u)
    y = u(1) | u(2);

== matlab function Control_Logic_b_chk2/NOT5/MATLAB Function ==
  data: u input; y output
%反転
function y = NOT(u)
    if u == false        
        y = true;
    else
        y = false;
    end

== matlab function Control_Logic_b_chk2/AND7/MATLAB Function ==
  data: u input; y output
% 論理積
function y = AND(u)
    y = u(1) & u(2);

== matlab function Control_Logic_b_chk2/AND8/MATLAB Function ==
  data: u input; y output
% 論理積
function y = AND(u)
    y = u(1) & u(2);

== matlab function Control_Logic_b_chk2/OSHOTC12/MATLAB Function ==
  data: u input; y output; w output; yold input; set input; timc input
% ワンショット タイマ
%  xがOFFからONに変化してからパラメータで設定した[sec]の間、yをONとする。
%  なお、xのON状態がパラメータで設定した[sec]以上継続した場合、あるいは設定以下
%  しか継続しない場合でも、yのON状態の期間はパラメータで設定した時間となる。
%       ud(1)：入力信号
%       yold：前回値
%       set：時定数
%       timc(1)：計算刻み
%       timc(2)：経過時間
%       y : 出力信号
function[y, w] = OSHOTC(u, yold, set, timc)
    if (u == false) && (yold == false)
        w = 0;
        y = false;
    else
        if set > timc(2)
            y = true;
            w = timc(2) + timc(1);
        else
            y = false;
            w = timc(2);
            if u == false
                w = 0;
            end
        end
    end

== matlab function Control_Logic_b_chk2/OSHOTC13/MATLAB Function ==
  data: u input; y output; w output; yold input; set input; timc input
% ワンショット タイマ
%  xがOFFからONに変化してからパラメータで設定した[sec]の間、yをONとする。
%  なお、xのON状態がパラメータで設定した[sec]以上継続した場合、あるいは設定以下
%  しか継続しない場合でも、yのON状態の期間はパラメータで設定した時間となる。
%       ud(1)：入力信号
%       yold：前回値
%       set：時定数
%       timc(1)：計算刻み
%       timc(2)：経過時間
%       y : 出力信号
function[y, w] = OSHOTC(u, yold, set, timc)
    if (u == false) && (yold == false)
        w = 0;
        y = false;
    else
        if set > timc(2)
            y = true;
            w = timc(2) + timc(1);
        else
            y = false;
            w = timc(2);
            if u == false
                w = 0;
            end
        end
    end

== matlab function Control_Logic_b_chk2/OSHOTC14/MATLAB Function ==
  data: u input; y output; w output; yold input; set input; timc input
% ワンショット タイマ
%  xがOFFからONに変化してからパラメータで設定した[sec]の間、yをONとする。
%  なお、xのON状態がパラメータで設定した[sec]以上継続した場合、あるいは設定以下
%  しか継続しない場合でも、yのON状態の期間はパラメータで設定した時間となる。
%       ud(1)：入力信号
%       yold：前回値
%       set：時定数
%       timc(1)：計算刻み
%       timc(2)：経過時間
%       y : 出力信号
function[y, w] = OSHOTC(u, yold, set, timc)
    if (u == false) && (yold == false)
        w = 0;
        y = false;
    else
        if set > timc(2)
            y = true;
            w = timc(2) + timc(1);
        else
            y = false;
            w = timc(2);
            if u == false
                w = 0;
            end
        end
    end

== matlab function Control_Logic_b_chk2/OR3L5/MATLAB Function ==
  data: u input; y output
%論理和
function y = OR3(u)
    y = u(1) | u(2) | u(3);

== matlab function Control_Logic_b_chk2/OR3L6/MATLAB Function ==
  data: u input; y output
%論理和
function y = OR3(u)
    y = u(1) | u(2) | u(3);

== matlab function Control_Logic_b_chk2/OR2/MATLAB Function ==
  data: u input; y output
%論理和
function y = OR(u)
    y = u(1) | u(2);

== matlab function Control_Logic_b_chk2/AND9/MATLAB Function ==
  data: u input; y output
% 論理積
function y = AND(u)
    y = u(1) & u(2);

== matlab function Control_Logic_b_chk2/AND10/MATLAB Function ==
  data: u input; y output
% 論理積
function y = AND(u)
    y = u(1) & u(2);

== matlab function Control_Logic_b_chk2/AND11/MATLAB Function ==
  data: u input; y output
% 論理積
function y = AND(u)
    y = u(1) & u(2);

== matlab function Control_Logic_b_chk2/AND12/MATLAB Function ==
  data: u input; y output
% 論理積
function y = AND(u)
    y = u(1) & u(2);

== matlab function Control_Logic_b_chk2/NOT6/MATLAB Function ==
  data: u input; y output
%反転
function y = NOT(u)
    if u == false        
        y = true;
    else
        y = false;
    end

== matlab function Control_Logic_b_chk2/NOT7/MATLAB Function ==
  data: u input; y output
%反転
function y = NOT(u)
    if u == false        
        y = true;
    else
        y = false;
    end

== matlab function Control_Logic_b_chk2/FF3/MATLAB Function ==
  data: yold input; y output; set input
% フリップフロップ
%  セット入力がONのとき、yはON
%  リセット入力がONのとき、yはOFF
%  セット入力、リセット入力共にONまたはOFFのときは前回値を保持
%       yold:前回値
%       set(1):セット信号
%       set(2)：リセット信号
%       y : 出力信号
function y = FF(yold, set)
    y = yold;
    if (set(1) == false) && (set(2) == true)
        y = false;
    else
        if (set(1) == true) && (set(2) == false)
            y = true;
        end
    end

== matlab function Control_Logic_b_chk2/FF4/MATLAB Function ==
  data: yold input; y output; set input
% フリップフロップ
%  セット入力がONのとき、yはON
%  リセット入力がONのとき、yはOFF
%  セット入力、リセット入力共にONまたはOFFのときは前回値を保持
%       yold:前回値
%       set(1):セット信号
%       set(2)：リセット信号
%       y : 出力信号
function y = FF(yold, set)
    y = yold;
    if (set(1) == false) && (set(2) == true)
        y = false;
    else
        if (set(1) == true) && (set(2) == false)
            y = true;
        end
    end

== matlab function Control_Logic_b_chk2/SUB/MATLAB Function ==
  data: u input; y output
% 減算器
function y = SUB(u)
    y = u(1) - u(2);

== matlab function Control_Logic_b_chk2/OSHOTC15/MATLAB Function ==
  data: u input; y output; w output; yold input; set input; timc input
% ワンショット タイマ
%  xがOFFからONに変化してからパラメータで設定した[sec]の間、yをONとする。
%  なお、xのON状態がパラメータで設定した[sec]以上継続した場合、あるいは設定以下
%  しか継続しない場合でも、yのON状態の期間はパラメータで設定した時間となる。
%       ud(1)：入力信号
%       yold：前回値
%       set：時定数
%       timc(1)：計算刻み
%       timc(2)：経過時間
%       y : 出力信号
function[y, w] = OSHOTC(u, yold, set, timc)
    if (u == false) && (yold == false)
        w = 0;
        y = false;
    else
        if set > timc(2)
            y = true;
            w = timc(2) + timc(1);
        else
            y = false;
            w = timc(2);
            if u == false
                w = 0;
            end
        end
    end

== matlab function Control_Logic_b_chk2/COMP/MATLAB Function ==
  data: u input; y output; set input
% 設定値比較
%   x≧Setならば、 yをON
%   x＜Setならば、 yをOFF
%       u : 入力変数
%       Set : 入力変数
%       y : 出力変数
function y = COMP(u, set)
    if u >= set
        y = true;
    else
        y = false; 
    end

== matlab function Control_Logic_b_chk2/ANSW/MATLAB Function ==
  data: ud input; y output; ua input
% 2位置(アナログ)スイッチ
%   C入力がONならば、 y=x1(A入力を選択)
%   C入力がOFFならば、 y=x2(B入力を選択)
%       ua(1):A入力変数
%       ua(2):B入力変数
%       ud:C入力変数
%       y : 出力変数
function y = ANSW(ud, ua)
    if ud ~= false
        y = ua(1);
    else
        y = ua(2); 
    end

== matlab function Control_Logic_b_chk2/ANSW1/MATLAB Function ==
  data: ud input; y output; ua input
% 2位置(アナログ)スイッチ
%   C入力がONならば、 y=x1(A入力を選択)
%   C入力がOFFならば、 y=x2(B入力を選択)
%       ua(1):A入力変数
%       ua(2):B入力変数
%       ud:C入力変数
%       y : 出力変数
function y = ANSW(ud, ua)
    if ud ~= false
        y = ua(1);
    else
        y = ua(2); 
    end

== matlab function Control_Logic_b_chk2/ANSW2/MATLAB Function ==
  data: ud input; y output; ua input
% 2位置(アナログ)スイッチ
%   C入力がONならば、 y=x1(A入力を選択)
%   C入力がOFFならば、 y=x2(B入力を選択)
%       ua(1):A入力変数
%       ua(2):B入力変数
%       ud:C入力変数
%       y : 出力変数
function y = ANSW(ud, ua)
    if ud ~= false
        y = ua(1);
    else
        y = ua(2); 
    end

== matlab function Control_Logic_b_chk2/ANSW3/MATLAB Function ==
  data: ud input; y output; ua input
% 2位置(アナログ)スイッチ
%   C入力がONならば、 y=x1(A入力を選択)
%   C入力がOFFならば、 y=x2(B入力を選択)
%       ua(1):A入力変数
%       ua(2):B入力変数
%       ud:C入力変数
%       y : 出力変数
function y = ANSW(ud, ua)
    if ud ~= false
        y = ua(1);
    else
        y = ua(2); 
    end

== matlab function Control_Logic_b_chk2/ANSW4/MATLAB Function ==
  data: ud input; y output; ua input
% 2位置(アナログ)スイッチ
%   C入力がONならば、 y=x1(A入力を選択)
%   C入力がOFFならば、 y=x2(B入力を選択)
%       ua(1):A入力変数
%       ua(2):B入力変数
%       ud:C入力変数
%       y : 出力変数
function y = ANSW(ud, ua)
    if ud ~= false
        y = ua(1);
    else
        y = ua(2); 
    end

== matlab function Control_Logic_b_chk2/ANSW5/MATLAB Function ==
  data: ud input; y output; ua input
% 2位置(アナログ)スイッチ
%   C入力がONならば、 y=x1(A入力を選択)
%   C入力がOFFならば、 y=x2(B入力を選択)
%       ua(1):A入力変数
%       ua(2):B入力変数
%       ud:C入力変数
%       y : 出力変数
function y = ANSW(ud, ua)
    if ud ~= false
        y = ua(1);
    else
        y = ua(2); 
    end

== matlab function Control_Logic_b_chk2/ANSW6/MATLAB Function ==
  data: ud input; y output; ua input
% 2位置(アナログ)スイッチ
%   C入力がONならば、 y=x1(A入力を選択)
%   C入力がOFFならば、 y=x2(B入力を選択)
%       ua(1):A入力変数
%       ua(2):B入力変数
%       ud:C入力変数
%       y : 出力変数
function y = ANSW(ud, ua)
    if ud ~= false
        y = ua(1);
    else
        y = ua(2); 
    end

== matlab function Control_Logic_b_chk2/Position control/SUB/MATLAB Function ==
  data: u input; y output
% 減算器
function y = SUB(u)
    y = u(1) - u(2);

== matlab function Control_Logic_b_chk2/Position control/MUL/MATLAB Function ==
  data: u input; y output
% 乗算器
function y = MUL(u)
    y = u(1) * u(2);

== matlab function Control_Logic_b_chk2/Position control/MUL1/MATLAB Function ==
  data: u input; y output
% 乗算器
function y = MUL(u)
    y = u(1) * u(2);

== matlab function Control_Logic_b_chk2/Position control/DIV/MATLAB Function ==
  data: u input; y output; err output; set input
% 除算器
%       u(1), u(2) : 入力変数
%       set : FloatMax
%       y : 出力変数
function [y, err] = DIV(u, set)
    y = set;
    err = -1;
    if u(2) ~= 0
        y = u(1) / u(2);
        err = 1;
    end

== matlab function Control_Logic_b_chk2/Position control/SUB1/MATLAB Function ==
  data: u input size=2; y output size=1
% 減算器
function y = SUB(u)
    y = u(1) - u(2);

== matlab function Control_Logic_b_chk2/Position control/SUB2/MATLAB Function ==
  data: u input; y output
% 減算器
function y = SUB(u)
    y = u(1) - u(2);

== matlab function Control_Logic_b_chk2/Position control/DIV1/MATLAB Function ==
  data: u input; y output; err output; set input
% 除算器
%       u(1), u(2) : 入力変数
%       set : FloatMax
%       y : 出力変数
function [y, err] = DIV(u, set)
    y = set;
    err = -1;
    if u(2) ~= 0
        y = u(1) / u(2);
        err = 1;
    end

== matlab function Control_Logic_b_chk2/Position control/SUB3/MATLAB Function ==
  data: u input; y output
% 減算器
function y = SUB(u)
    y = u(1) - u(2);

== matlab function Control_Logic_b_chk2/Position control/HSS/MATLAB Function ==
  data: u input; y output
% 高値選択器
function y = HSS(u)
    y = u(1);
    if u(2) > y 
        y = u(2);
    end

== matlab function Control_Logic_b_chk2/Position control/LSS/MATLAB Function ==
  data: u input; y output
% 低値選択器
function y = LSS(u)
    y = u(1);
    if u(2) < y 
        y = u(2);
    end

== matlab function Control_Logic_b_chk2/Velocity control/DIV/MATLAB Function ==
  data: u input; y output; err output; set input
% 除算器
%       u(1), u(2) : 入力変数
%       set : FloatMax
%       y : 出力変数
function [y, err] = DIV(u, set)
    y = set;
    err = -1;
    if u(2) ~= 0
        y = u(1) / u(2);
        err = 1;
    end

== matlab function Control_Logic_b_chk2/Velocity control/MUL/MATLAB Function ==
  data: u input; y output
% 乗算器
function y = MUL(u)
    y = u(1) * u(2);
